simulink model "Thirtybussys1"  (R2021a)
settings: Solver=VariableStepAuto  StartTime=0.0  StopTime=4.0  RelTol=1e-3
libraries: spsFourierLib x60, spsThreePhaseSeriesRLCBranchLib x41, spsThreePhaseVIMeasurementLib x30, spsThreePhaseSeriesRLCLoadLib x21, spsThreePhaseSourceLib x6, spsThreePhaseTransformerTwoWindingsLib x6, spsThreePhaseFaultLib x2, spspowerguiLib x1
(part 1 of 2)
settings Model: Creator=sariy sh  LastModifiedBy=Maruf
settings SolverCC: AlgebraicLoopSolver=TrustRegion
settings DataIOCC: ReturnWorkspaceOutputs=off
settings DebuggingCC: SFMachineParentedDataDiag=warning  ArithmeticOperatorsInVariantConditions=warning
settings SFSimCC: SimUseLocalCustomCode=off  CustomCodeUndefinedFunction=UseInterfaceOnly
settings RTWCC: RTWUseLocalCustomCode=off
settings CodeAppCC: StateflowObjectComments=on
settings SimscapeCC: SimscapeNormalizeSystem=off

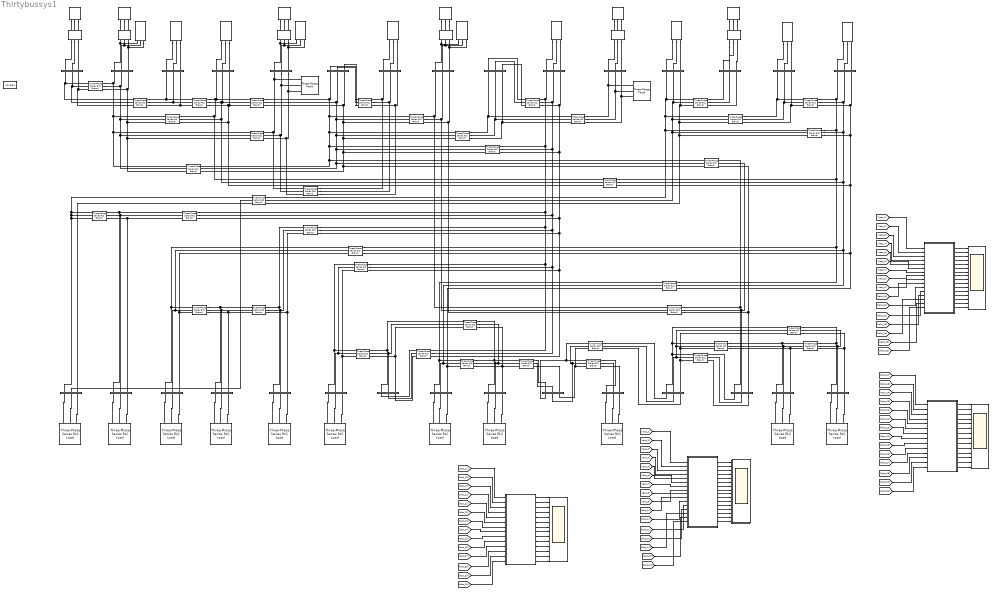
== system Thirtybussys1 ==
  3-Phase Fault : spsThreePhaseFaultLib/Three-Phase Fault  InitialStates=0  FaultA=on  FaultB=on  FaultC=on  GroundFault=on  SwitchTimes=[2.1 3.1]  External=off  SwitchStatus=NaN  FaultResistance=0.01  GroundResistance=0.001  SnubberResistance=1e6  SnubberCapacitance=inf  Measurements=Fault currents
  3-Phase Fault1 : spsThreePhaseFaultLib/Three-Phase Fault  InitialStates=0  FaultA=on  FaultB=on  FaultC=on  GroundFault=on  SwitchTimes=[2.1 3.1]  External=off  SwitchStatus=NaN  FaultResistance=0.01  GroundResistance=0.001  SnubberResistance=1e6  SnubberCapacitance=inf  Measurements=Fault currents
  Bus 1 : spsThreePhaseVIMeasurementLib/Three-Phase V-I Measurement  VoltageMeasurement=phase-to-ground  SetLabelV=on  LabelV=Vabc_1  Vpu=on  VpuLL=off  CurrentMeasurement=yes  SetLabelI=on  LabelI=Iabc_1  Ipu=on  Pbase=100e6  Vbase=500e3  OutputType=Complex  PhasorSimulation=off  PSBequivalent=0
  Bus 10 : spsThreePhaseVIMeasurementLib/Three-Phase V-I Measurement  VoltageMeasurement=phase-to-ground  SetLabelV=on  LabelV=Vabc_10  Vpu=on  VpuLL=off  CurrentMeasurement=yes  SetLabelI=on  LabelI=Iabc_10  Ipu=on  Pbase=100e6  Vbase=500e3  OutputType=Complex  PhasorSimulation=off  PSBequivalent=0
  Bus 11 : spsThreePhaseVIMeasurementLib/Three-Phase V-I Measurement  VoltageMeasurement=phase-to-ground  SetLabelV=on  LabelV=Vabc_11  Vpu=on  VpuLL=off  CurrentMeasurement=yes  SetLabelI=on  LabelI=Iabc_11  Ipu=on  Pbase=100e6  Vbase=500e3  OutputType=Complex  PhasorSimulation=off  PSBequivalent=0
  Bus 12 : spsThreePhaseVIMeasurementLib/Three-Phase V-I Measurement  VoltageMeasurement=phase-to-ground  SetLabelV=on  LabelV=Vabc_12  Vpu=on  VpuLL=off  CurrentMeasurement=yes  SetLabelI=on  LabelI=Iabc_12  Ipu=on  Pbase=100e6  Vbase=500e3  OutputType=Complex  PhasorSimulation=off  PSBequivalent=0
  Bus 13 : spsThreePhaseVIMeasurementLib/Three-Phase V-I Measurement  VoltageMeasurement=phase-to-ground  SetLabelV=on  LabelV=Vabc_13  Vpu=on  VpuLL=off  CurrentMeasurement=yes  SetLabelI=on  LabelI=Iabc_13  Ipu=on  Pbase=100e6  Vbase=500e3  OutputType=Complex  PhasorSimulation=off  PSBequivalent=0
  Bus 14 : spsThreePhaseVIMeasurementLib/Three-Phase V-I Measurement  VoltageMeasurement=phase-to-ground  SetLabelV=on  LabelV=Vabc_14  Vpu=on  VpuLL=off  CurrentMeasurement=yes  SetLabelI=on  LabelI=Iabc_14  Ipu=on  Pbase=100e6  Vbase=500e3  OutputType=Complex  PhasorSimulation=off  PSBequivalent=0
  Bus 15 : spsThreePhaseVIMeasurementLib/Three-Phase V-I Measurement  VoltageMeasurement=phase-to-ground  SetLabelV=on  LabelV=Vabc_15  Vpu=on  VpuLL=off  CurrentMeasurement=yes  SetLabelI=on  LabelI=Iabc_15  Ipu=on  Pbase=100e6  Vbase=500e3  OutputType=Complex  PhasorSimulation=off  PSBequivalent=0
  Bus 16 : spsThreePhaseVIMeasurementLib/Three-Phase V-I Measurement  VoltageMeasurement=phase-to-ground  SetLabelV=on  LabelV=Vabc_16  Vpu=on  VpuLL=off  CurrentMeasurement=yes  SetLabelI=on  LabelI=Iabc_16  Ipu=on  Pbase=100e6  Vbase=500e3  OutputType=Complex  PhasorSimulation=off  PSBequivalent=0
  Bus 17 : spsThreePhaseVIMeasurementLib/Three-Phase V-I Measurement  VoltageMeasurement=phase-to-ground  SetLabelV=on  LabelV=Vabc_17  Vpu=on  VpuLL=off  CurrentMeasurement=yes  SetLabelI=on  LabelI=Iabc_17  Ipu=on  Pbase=100e6  Vbase=500e3  OutputType=Complex  PhasorSimulation=off  PSBequivalent=0
  Bus 18 : spsThreePhaseVIMeasurementLib/Three-Phase V-I Measurement  VoltageMeasurement=phase-to-ground  SetLabelV=on  LabelV=Vabc_18  Vpu=on  VpuLL=off  CurrentMeasurement=yes  SetLabelI=on  LabelI=Iabc_18  Ipu=on  Pbase=100e6  Vbase=500e3  OutputType=Complex  PhasorSimulation=off  PSBequivalent=0
  Bus 19 : spsThreePhaseVIMeasurementLib/Three-Phase V-I Measurement  VoltageMeasurement=phase-to-ground  SetLabelV=on  LabelV=Vabc_19  Vpu=on  VpuLL=off  CurrentMeasurement=yes  SetLabelI=on  LabelI=Iabc_19  Ipu=on  Pbase=100e6  Vbase=500e3  OutputType=Complex  PhasorSimulation=off  PSBequivalent=0
  Bus 2 : spsThreePhaseVIMeasurementLib/Three-Phase V-I Measurement  VoltageMeasurement=phase-to-ground  SetLabelV=on  LabelV=Vabc_2  Vpu=on  VpuLL=off  CurrentMeasurement=yes  SetLabelI=on  LabelI=Iabc_2  Ipu=on  Pbase=100e6  Vbase=500e3  OutputType=Complex  PhasorSimulation=off  PSBequivalent=0
  Bus 20 : spsThreePhaseVIMeasurementLib/Three-Phase V-I Measurement  VoltageMeasurement=phase-to-ground  SetLabelV=on  LabelV=Vabc_20  Vpu=on  VpuLL=off  CurrentMeasurement=yes  SetLabelI=on  LabelI=Iabc_20  Ipu=on  Pbase=100e6  Vbase=500e3  OutputType=Complex  PhasorSimulation=off  PSBequivalent=0
  Bus 21 : spsThreePhaseVIMeasurementLib/Three-Phase V-I Measurement  VoltageMeasurement=phase-to-ground  SetLabelV=on  LabelV=Vabc_21  Vpu=on  VpuLL=off  CurrentMeasurement=yes  SetLabelI=on  LabelI=Iabc_21  Ipu=on  Pbase=100e6  Vbase=500e3  OutputType=Complex  PhasorSimulation=off  PSBequivalent=0
  Bus 22 : spsThreePhaseVIMeasurementLib/Three-Phase V-I Measurement  VoltageMeasurement=phase-to-ground  SetLabelV=on  LabelV=Vabc_22  Vpu=on  VpuLL=off  CurrentMeasurement=yes  SetLabelI=on  LabelI=Iabc_22  Ipu=on  Pbase=100e6  Vbase=500e3  OutputType=Complex  PhasorSimulation=off  PSBequivalent=0
  Bus 23 : spsThreePhaseVIMeasurementLib/Three-Phase V-I Measurement  VoltageMeasurement=phase-to-ground  SetLabelV=on  LabelV=Vabc_23  Vpu=on  VpuLL=off  CurrentMeasurement=yes  SetLabelI=on  LabelI=Iabc_23  Ipu=on  Pbase=100e6  Vbase=500e3  OutputType=Complex  PhasorSimulation=off  PSBequivalent=0
  Bus 24 : spsThreePhaseVIMeasurementLib/Three-Phase V-I Measurement  VoltageMeasurement=phase-to-ground  SetLabelV=on  LabelV=Vabc_24  Vpu=on  VpuLL=off  CurrentMeasurement=yes  SetLabelI=on  LabelI=Iabc_24  Ipu=on  Pbase=100e6  Vbase=500e3  OutputType=Complex  PhasorSimulation=off  PSBequivalent=0
  Bus 25 : spsThreePhaseVIMeasurementLib/Three-Phase V-I Measurement  VoltageMeasurement=phase-to-ground  SetLabelV=on  LabelV=Vabc_25  Vpu=on  VpuLL=off  CurrentMeasurement=yes  SetLabelI=on  LabelI=Iabc_25  Ipu=on  Pbase=100e6  Vbase=500e3  OutputType=Complex  PhasorSimulation=off  PSBequivalent=0
  Bus 26 : spsThreePhaseVIMeasurementLib/Three-Phase V-I Measurement  VoltageMeasurement=phase-to-ground  SetLabelV=on  LabelV=Vabc_26  Vpu=on  VpuLL=off  CurrentMeasurement=yes  SetLabelI=on  LabelI=Iabc_26  Ipu=on  Pbase=100e6  Vbase=500e3  OutputType=Complex  PhasorSimulation=off  PSBequivalent=0
  Bus 27 : spsThreePhaseVIMeasurementLib/Three-Phase V-I Measurement  VoltageMeasurement=phase-to-ground  SetLabelV=on  LabelV=Vabc_27  Vpu=on  VpuLL=off  CurrentMeasurement=yes  SetLabelI=on  LabelI=Iabc_27  Ipu=on  Pbase=100e6  Vbase=500e3  OutputType=Complex  PhasorSimulation=off  PSBequivalent=0
  Bus 28 : spsThreePhaseVIMeasurementLib/Three-Phase V-I Measurement  VoltageMeasurement=phase-to-ground  SetLabelV=on  LabelV=Vabc_28  Vpu=on  VpuLL=off  CurrentMeasurement=yes  SetLabelI=on  LabelI=Iabc_28  Ipu=on  Pbase=100e6  Vbase=500e3  OutputType=Complex  PhasorSimulation=off  PSBequivalent=0
  Bus 29 : spsThreePhaseVIMeasurementLib/Three-Phase V-I Measurement  VoltageMeasurement=phase-to-ground  SetLabelV=on  LabelV=Vabc_29  Vpu=on  VpuLL=off  CurrentMeasurement=yes  SetLabelI=on  LabelI=Iabc_29  Ipu=on  Pbase=100e6  Vbase=500e3  OutputType=Complex  PhasorSimulation=off  PSBequivalent=0
  Bus 3 : spsThreePhaseVIMeasurementLib/Three-Phase V-I Measurement  VoltageMeasurement=phase-to-ground  SetLabelV=on  LabelV=Vabc_3  Vpu=on  VpuLL=off  CurrentMeasurement=yes  SetLabelI=on  LabelI=Iabc_3  Ipu=on  Pbase=100e6  Vbase=500e3  OutputType=Complex  PhasorSimulation=off  PSBequivalent=0
  Bus 30 : spsThreePhaseVIMeasurementLib/Three-Phase V-I Measurement  VoltageMeasurement=phase-to-ground  SetLabelV=on  LabelV=Vabc_30  Vpu=on  VpuLL=off  CurrentMeasurement=yes  SetLabelI=on  LabelI=Iabc_30  Ipu=on  Pbase=100e6  Vbase=500e3  OutputType=Complex  PhasorSimulation=off  PSBequivalent=0
  Bus 4 : spsThreePhaseVIMeasurementLib/Three-Phase V-I Measurement  VoltageMeasurement=phase-to-ground  SetLabelV=on  LabelV=Vabc_4  Vpu=on  VpuLL=off  CurrentMeasurement=yes  SetLabelI=on  LabelI=Iabc_4  Ipu=on  Pbase=100e6  Vbase=500e3  OutputType=Complex  PhasorSimulation=off  PSBequivalent=0
  Bus 5 : spsThreePhaseVIMeasurementLib/Three-Phase V-I Measurement  VoltageMeasurement=phase-to-ground  SetLabelV=on  LabelV=Vabc_5  Vpu=on  VpuLL=off  CurrentMeasurement=yes  SetLabelI=on  LabelI=Iabc_5  Ipu=on  Pbase=100e6  Vbase=500e3  OutputType=Complex  PhasorSimulation=off  PSBequivalent=0
  Bus 6 : spsThreePhaseVIMeasurementLib/Three-Phase V-I Measurement  VoltageMeasurement=phase-to-ground  SetLabelV=on  LabelV=Vabc_6  Vpu=on  VpuLL=off  CurrentMeasurement=yes  SetLabelI=on  LabelI=Iabc_6  Ipu=on  Pbase=100e6  Vbase=500e3  OutputType=Complex  PhasorSimulation=off  PSBequivalent=0
  Bus 7 : spsThreePhaseVIMeasurementLib/Three-Phase V-I Measurement  VoltageMeasurement=phase-to-ground  SetLabelV=on  LabelV=Vabc_7  Vpu=on  VpuLL=off  CurrentMeasurement=yes  SetLabelI=on  LabelI=Iabc_7  Ipu=on  Pbase=100e6  Vbase=500e3  OutputType=Complex  PhasorSimulation=off  PSBequivalent=0
  Bus 8 : spsThreePhaseVIMeasurementLib/Three-Phase V-I Measurement  VoltageMeasurement=phase-to-ground  SetLabelV=on  LabelV=Vabc_8  Vpu=on  VpuLL=off  CurrentMeasurement=yes  SetLabelI=on  LabelI=Iabc_8  Ipu=on  Pbase=100e6  Vbase=500e3  OutputType=Complex  PhasorSimulation=off  PSBequivalent=0
  Bus 9 : spsThreePhaseVIMeasurementLib/Three-Phase V-I Measurement  VoltageMeasurement=phase-to-ground  SetLabelV=on  LabelV=Vabc_9  Vpu=on  VpuLL=off  CurrentMeasurement=yes  SetLabelI=on  LabelI=Iabc_9  Ipu=on  Pbase=100e6  Vbase=500e3  OutputType=Complex  PhasorSimulation=off  PSBequivalent=0
  Gen1 : spsThreePhaseSourceLib/Three-Phase Source  InternalConnection=Yg  VoltagePhases=off  Voltage=1.06  PhaseAngle=0  Voltage_phases=[25e3 25e3 25e3]/sqrt(3)  PhaseAngles_phases=[0 -120 +120]  Frequency=50  NonIdealSource=on  SpecifyImpedance=on  Resistance=0.8929  Inductance=16.58e-3  ShortCircuitLevel=100e6  BaseVoltage=1  XRratio=1  BusType=swing  Pref=10e3  Qref=0  Prefabc=[10e3, 10e3, 10e3]  Qrefabc=[0, 0, 0]  Qmin=-inf  Qmax=inf
  Gen2 : spsThreePhaseSourceLib/Three-Phase Source  InternalConnection=Yg  VoltagePhases=off  Voltage=1.045  PhaseAngle=0  Voltage_phases=[25e3 25e3 25e3]/sqrt(3)  PhaseAngles_phases=[0 -120 +120]  Frequency=50  NonIdealSource=on  SpecifyImpedance=on  Resistance=0.8929  Inductance=16.58e-3  ShortCircuitLevel=100e6  BaseVoltage=1  XRratio=1  BusType=PQ  Pref=0.4  Qref=0.5  Prefabc=[10e3, 10e3, 10e3]  Qrefabc=[0, 0, 0]  Qmin=-inf  Qmax=inf
  Gen3 : spsThreePhaseSourceLib/Three-Phase Source  InternalConnection=Yg  VoltagePhases=off  Voltage=1.010  PhaseAngle=0  Voltage_phases=[25e3 25e3 25e3]/sqrt(3)  PhaseAngles_phases=[0 -120 +120]  Frequency=50  NonIdealSource=on  SpecifyImpedance=on  Resistance=0.8929  Inductance=16.58e-3  ShortCircuitLevel=100e6  BaseVoltage=1  XRratio=1  BusType=PV  Pref=0.37  Qref=0  Prefabc=[10e3, 10e3, 10e3]  Qrefabc=[0, 0, 0]  Qmin=-0.15  Qmax=0.625
  Gen4 : spsThreePhaseSourceLib/Three-Phase Source  InternalConnection=Yg  VoltagePhases=off  Voltage=1.010  PhaseAngle=0  Voltage_phases=[25e3 25e3 25e3]/sqrt(3)  PhaseAngles_phases=[0 -120 +120]  Frequency=50  NonIdealSource=on  SpecifyImpedance=on  Resistance=0.8929  Inductance=16.58e-3  ShortCircuitLevel=100e6  BaseVoltage=1  XRratio=1  BusType=PV  Pref=0.373  Qref=0  Prefabc=[10e3, 10e3, 10e3]  Qrefabc=[0, 0, 0]  Qmin=-0.15  Qmax=0.50
  Gen5 : spsThreePhaseSourceLib/Three-Phase Source  InternalConnection=Yg  VoltagePhases=off  Voltage=1.082  PhaseAngle=0  Voltage_phases=[25e3 25e3 25e3]/sqrt(3)  PhaseAngles_phases=[0 -120 +120]  Frequency=50  NonIdealSource=on  SpecifyImpedance=on  Resistance=0.8929  Inductance=16.58e-3  ShortCircuitLevel=100e6  BaseVoltage=1  XRratio=1  BusType=PV  Pref=0.162  Qref=0  Prefabc=[10e3, 10e3, 10e3]  Qrefabc=[0, 0, 0]  Qmin=-0.10  Qmax=0.40
  Gen6 : spsThreePhaseSourceLib/Three-Phase Source  InternalConnection=Yg  VoltagePhases=off  Voltage=1.071  PhaseAngle=0  Voltage_phases=[25e3 25e3 25e3]/sqrt(3)  PhaseAngles_phases=[0 -120 +120]  Frequency=50  NonIdealSource=on  SpecifyImpedance=on  Resistance=0.8929  Inductance=16.58e-3  ShortCircuitLevel=100e6  BaseVoltage=1  XRratio=1  BusType=PV  Pref=0.106  Qref=0  Prefabc=[10e3, 10e3, 10e3]  Qrefabc=[0, 0, 0]  Qmin=-0.15  Qmax=0.45
  Scope1 : Scope  NumInputPorts=14
  Scope2 : Scope  NumInputPorts=16
  Scope3 : Scope  NumInputPorts=16
  Scope4 : Scope  NumInputPorts=14
  Scope5 : Scope  NumInputPorts=16
  Subsystem : Subsystem
  Subsystem1 : Subsystem
  Subsystem2 : Subsystem
  Subsystem3 : Subsystem
  Three-Phase Series RLC Branch : spsThreePhaseSeriesRLCBranchLib/Three-Phase Series RLC Branch  LConnTagsString=A|B|C  RConnTagsString=A|B|C  BranchType=RLC  Resistance=0.0192  Inductance=0.0575/(2*pi*50)  Capacitance=1/0.0264/(2*pi*50)  Measurements=None
  Three-Phase Series RLC Branch1 : spsThreePhaseSeriesRLCBranchLib/Three-Phase Series RLC Branch  LConnTagsString=A|B|C  RConnTagsString=A|B|C  BranchType=RLC  Resistance=0.0452  Inductance=0.1652/(2*pi*50)  Capacitance=1/0.0204/(2*pi*50)  Measurements=None
  Three-Phase Series RLC Branch10 : spsThreePhaseSeriesRLCBranchLib/Three-Phase Series RLC Branch  LConnTagsString=A|B|C  RConnTagsString=A|B|C  BranchType=L  Resistance=0  Inductance=0.2080/(2*pi*50)  Capacitance=0  Measurements=None
  Three-Phase Series RLC Branch11 : spsThreePhaseSeriesRLCBranchLib/Three-Phase Series RLC Branch  LConnTagsString=A|B|C  RConnTagsString=A|B|C  BranchType=L  Resistance=1  Inductance=0.1100/(2*pi*50)  Capacitance=1e-6  Measurements=None
  Three-Phase Series RLC Branch12 : spsThreePhaseSeriesRLCBranchLib/Three-Phase Series RLC Branch  LConnTagsString=A|B|C  RConnTagsString=A|B|C  BranchType=L  Resistance=1  Inductance=0.5560/(2*pi*50)  Capacitance=1e-6  Measurements=None
  Three-Phase Series RLC Branch13 : spsThreePhaseSeriesRLCBranchLib/Three-Phase Series RLC Branch  LConnTagsString=A|B|C  RConnTagsString=A|B|C  BranchType=L  Resistance=1  Inductance=0.2080/(2*pi*50)  Capacitance=1e-6  Measurements=None
  Three-Phase Series RLC Branch14 : spsThreePhaseSeriesRLCBranchLib/Three-Phase Series RLC Branch  LConnTagsString=A|B|C  RConnTagsString=A|B|C  BranchType=L  Resistance=1  Inductance=0.1400/(2*pi*50)  Capacitance=1e-6  Measurements=None
  Three-Phase Series RLC Branch15 : spsThreePhaseSeriesRLCBranchLib/Three-Phase Series RLC Branch  LConnTagsString=A|B|C  RConnTagsString=A|B|C  BranchType=RL  Resistance=0.1231  Inductance=0.2559/(2*pi*50)  Capacitance=1e-6  Measurements=None
  Three-Phase Series RLC Branch16 : spsThreePhaseSeriesRLCBranchLib/Three-Phase Series RLC Branch  LConnTagsString=A|B|C  RConnTagsString=A|B|C  BranchType=RL  Resistance=0.2210  Inductance=0.1997/(2*pi*50)  Capacitance=1e-6  Measurements=None
  Three-Phase Series RLC Branch17 : spsThreePhaseSeriesRLCBranchLib/Three-Phase Series RLC Branch  LConnTagsString=A|B|C  RConnTagsString=A|B|C  BranchType=L  Resistance=1  Inductance=0.2560/(2*pi*50)  Capacitance=1e-6  Measurements=None
  Three-Phase Series RLC Branch18 : spsThreePhaseSeriesRLCBranchLib/Three-Phase Series RLC Branch  LConnTagsString=A|B|C  RConnTagsString=A|B|C  BranchType=RL  Resistance=0.0945  Inductance=0.1987/(2*pi*50)  Capacitance=1e-6  Measurements=None
  Three-Phase Series RLC Branch19 : spsThreePhaseSeriesRLCBranchLib/Three-Phase Series RLC Branch  LConnTagsString=A|B|C  RConnTagsString=A|B|C  BranchType=RLC  Resistance=0.0524  Inductance=0.1923/(2*pi*50)  Capacitance=1e-6  Measurements=None
  Three-Phase Series RLC Branch2 : spsThreePhaseSeriesRLCBranchLib/Three-Phase Series RLC Branch  LConnTagsString=A|B|C  RConnTagsString=A|B|C  BranchType=RLC  Resistance=0.0132  Inductance=0.0379/(2*pi*50)  Capacitance=1/0.0042/(2*pi*50)  Measurements=None
  Three-Phase Series RLC Branch20 : spsThreePhaseSeriesRLCBranchLib/Three-Phase Series RLC Branch  LConnTagsString=A|B|C  RConnTagsString=A|B|C  BranchType=RL  Resistance=0.0324  Inductance=0.0845/(2*pi*50)  Capacitance=1e-6  Measurements=None
  Three-Phase Series RLC Branch21 : spsThreePhaseSeriesRLCBranchLib/Three-Phase Series RLC Branch  LConnTagsString=A|B|C  RConnTagsString=A|B|C  BranchType=RL  Resistance=0.1063  Inductance=0.2185/(2*pi*50)  Capacitance=1e-6  Measurements=None
  Three-Phase Series RLC Branch22 : spsThreePhaseSeriesRLCBranchLib/Three-Phase Series RLC Branch  LConnTagsString=A|B|C  RConnTagsString=A|B|C  BranchType=RL  Resistance=0.0639  Inductance=0.1292/(2*pi*50)  Capacitance=1e-6  Measurements=None
  Three-Phase Series RLC Branch23 : spsThreePhaseSeriesRLCBranchLib/Three-Phase Series RLC Branch  LConnTagsString=A|B|C  RConnTagsString=A|B|C  BranchType=RL  Resistance=0.0340  Inductance=0.0680/(2*pi*50)  Capacitance=1e-6  Measurements=None
  Three-Phase Series RLC Branch24 : spsThreePhaseSeriesRLCBranchLib/Three-Phase Series RLC Branch  LConnTagsString=A|B|C  RConnTagsString=A|B|C  BranchType=RL  Resistance=0.0936  Inductance=0.2090/(2*pi*50)  Capacitance=1e-6  Measurements=None
  Three-Phase Series RLC Branch25 : spsThreePhaseSeriesRLCBranchLib/Three-Phase Series RLC Branch  LConnTagsString=A|B|C  RConnTagsString=A|B|C  BranchType=RL  Resistance=0.0348  Inductance=0.0749/(2*pi*50)  Capacitance=1e-6  Measurements=None
  Three-Phase Series RLC Branch26 : spsThreePhaseSeriesRLCBranchLib/Three-Phase Series RLC Branch  LConnTagsString=A|B|C  RConnTagsString=A|B|C  BranchType=RL  Resistance=0.0116  Inductance=0.0236/(2*pi*50)  Capacitance=1e-6  Measurements=None
  Three-Phase Series RLC Branch27 : spsThreePhaseSeriesRLCBranchLib/Three-Phase Series RLC Branch  LConnTagsString=A|B|C  RConnTagsString=A|B|C  BranchType=RL  Resistance=0.0727  Inductance=0.1499/(2*pi*50)  Capacitance=1e-6  Measurements=None
  Three-Phase Series RLC Branch28 : spsThreePhaseSeriesRLCBranchLib/Three-Phase Series RLC Branch  LConnTagsString=A|B|C  RConnTagsString=A|B|C  BranchType=RL  Resistance=0.1000  Inductance=0.2020/(2*pi*50)  Capacitance=1e-6  Measurements=None
  Three-Phase Series RLC Branch29 : spsThreePhaseSeriesRLCBranchLib/Three-Phase Series RLC Branch  LConnTagsString=A|B|C  RConnTagsString=A|B|C  BranchType=RL  Resistance=0.1150  Inductance=0.1790/(2*pi*50)  Capacitance=1e-6  Measurements=None
  Three-Phase Series RLC Branch3 : spsThreePhaseSeriesRLCBranchLib/Three-Phase Series RLC Branch  LConnTagsString=A|B|C  RConnTagsString=A|B|C  BranchType=RLC  Resistance=0.0570  Inductance=0.1737/(2*pi*50)  Capacitance=1/0.0184/(2*pi*50)  Measurements=None
  Three-Phase Series RLC Branch30 : spsThreePhaseSeriesRLCBranchLib/Three-Phase Series RLC Branch  LConnTagsString=A|B|C  RConnTagsString=A|B|C  BranchType=RL  Resistance=0.1320  Inductance=0.2700/(2*pi*50)  Capacitance=1e-6  Measurements=None
  Three-Phase Series RLC Branch31 : spsThreePhaseSeriesRLCBranchLib/Three-Phase Series RLC Branch  LConnTagsString=A|B|C  RConnTagsString=A|B|C  BranchType=RL  Resistance=0.1885  Inductance=0.3292/(2*pi*50)  Capacitance=1e-6  Measurements=None
  Three-Phase Series RLC Branch32 : spsThreePhaseSeriesRLCBranchLib/Three-Phase Series RLC Branch  LConnTagsString=A|B|C  RConnTagsString=A|B|C  BranchType=RL  Resistance=0.2544  Inductance=0.3800/(2*pi*50)  Capacitance=1e-6  Measurements=None
  Three-Phase Series RLC Branch33 : spsThreePhaseSeriesRLCBranchLib/Three-Phase Series RLC Branch  LConnTagsString=A|B|C  RConnTagsString=A|B|C  BranchType=RL  Resistance=0.1093  Inductance=0.2087/(2*pi*50)  Capacitance=1e-6  Measurements=None
  Three-Phase Series RLC Branch34 : spsThreePhaseSeriesRLCBranchLib/Three-Phase Series RLC Branch  LConnTagsString=A|B|C  RConnTagsString=A|B|C  BranchType=RL  Resistance=0.2198  Inductance=0.4153/(2*pi*50)  Capacitance=1e-6  Measurements=None
  Three-Phase Series RLC Branch35 : spsThreePhaseSeriesRLCBranchLib/Three-Phase Series RLC Branch  LConnTagsString=A|B|C  RConnTagsString=A|B|C  BranchType=RL  Resistance=0.3202  Inductance=0.6027/(2*pi*50)  Capacitance=1e-6  Measurements=None
  Three-Phase Series RLC Branch36 : spsThreePhaseSeriesRLCBranchLib/Three-Phase Series RLC Branch  LConnTagsString=A|B|C  RConnTagsString=A|B|C  BranchType=L  Resistance=1  Inductance=0.3960/(2*pi*50)  Capacitance=1e-6  Measurements=None
  Three-Phase Series RLC Branch37 : spsThreePhaseSeriesRLCBranchLib/Three-Phase Series RLC Branch  LConnTagsString=A|B|C  RConnTagsString=A|B|C  BranchType=RLC  Resistance=0.0169  Inductance=0.0599/(2*pi*50)  Capacitance=1/0.0065/(2*pi*50)  Measurements=None
  Three-Phase Series RLC Branch38 : spsThreePhaseSeriesRLCBranchLib/Three-Phase Series RLC Branch  LConnTagsString=A|B|C  RConnTagsString=A|B|C  BranchType=RLC  Resistance=0.0636  Inductance=0.2000/(2*pi*50)  Capacitance=1/0.0214/(2*pi*50)  Measurements=None
  Three-Phase Series RLC Branch39 : spsThreePhaseSeriesRLCBranchLib/Three-Phase Series RLC Branch  LConnTagsString=A|B|C  RConnTagsString=A|B|C  BranchType=RL  Resistance=0.0662  Inductance=0.1304/(2*pi*50)  Capacitance=1e-6  Measurements=None
  Three-Phase Series RLC Branch4 : spsThreePhaseSeriesRLCBranchLib/Three-Phase Series RLC Branch  LConnTagsString=A|B|C  RConnTagsString=A|B|C  BranchType=RLC  Resistance=0.0472  Inductance=0.1983/(2*pi*50)  Capacitance=1/0.0209/(2*pi*50)  Measurements=None
  Three-Phase Series RLC Branch40 : spsThreePhaseSeriesRLCBranchLib/Three-Phase Series RLC Branch  LConnTagsString=A|B|C  RConnTagsString=A|B|C  BranchType=RL  Resistance=0.2399  Inductance=0.4533/(2*pi*50)  Capacitance=1e-6  Measurements=None
  Three-Phase Series RLC Branch5 : spsThreePhaseSeriesRLCBranchLib/Three-Phase Series RLC Branch  LConnTagsString=A|B|C  RConnTagsString=A|B|C  BranchType=RLC  Resistance=0.0581  Inductance=0.1763/(2*pi*50)  Capacitance=1/0.0187/(2*pi*50)  Measurements=None
  Three-Phase Series RLC Branch6 : spsThreePhaseSeriesRLCBranchLib/Three-Phase Series RLC Branch  LConnTagsString=A|B|C  RConnTagsString=A|B|C  BranchType=RLC  Resistance=0.0119  Inductance=0.0414/(2*pi*50)  Capacitance=1/0.0045/(2*pi*50)  Measurements=None
  Three-Phase Series RLC Branch7 : spsThreePhaseSeriesRLCBranchLib/Three-Phase Series RLC Branch  LConnTagsString=A|B|C  RConnTagsString=A|B|C  BranchType=RLC  Resistance=0.0267  Inductance=0.0820/(2*pi*50)  Capacitance=1/0.0085/(2*pi*50)  Measurements=None
  Three-Phase Series RLC Branch8 : spsThreePhaseSeriesRLCBranchLib/Three-Phase Series RLC Branch  LConnTagsString=A|B|C  RConnTagsString=A|B|C  BranchType=RLC  Resistance=0.0460  Inductance=0.1160/(2*pi*50)  Capacitance=1/0.0102/(2*pi*50)  Measurements=None
  Three-Phase Series RLC Branch9 : spsThreePhaseSeriesRLCBranchLib/Three-Phase Series RLC Branch  LConnTagsString=A|B|C  RConnTagsString=A|B|C  BranchType=RLC  Resistance=0.0120  Inductance=0.0420/(2*pi*50)  Capacitance=1/0.0045/(2*pi*50)  Measurements=None
  Three-Phase Series RLC Load : spsThreePhaseSeriesRLCLoadLib/Three-Phase Series RLC Load  LConnTagsString=A|B|C  Configuration=Y (grounded)  NominalVoltage=1  Vabc=[1e3 1e3 1e3]  Vabcp=[1e3 1e3 1e3]  NominalFrequency=50  UnbalancedPower=off  ActivePower=0.217  InductivePower=0.127  CapacitivePower=0  Pabc=[10e3 9e3 11e3]  QLabc=[100 90 110]  QCabc=[100 90 110]  Pabcp=[10e3 9e3 11e3]  QLabcp=[100 90 110]  QCabcp=[100 90 110]  Measurements=None  LoadType=constant Z
  Three-Phase Series RLC Load1 : spsThreePhaseSeriesRLCLoadLib/Three-Phase Series RLC Load  LConnTagsString=A|B|C  Configuration=Y (grounded)  NominalVoltage=1  Vabc=[1e3 1e3 1e3]  Vabcp=[1e3 1e3 1e3]  NominalFrequency=50  UnbalancedPower=off  ActivePower=0.024  InductivePower=0.012  CapacitivePower=0  Pabc=[10e3 9e3 11e3]  QLabc=[100 90 110]  QCabc=[100 90 110]  Pabcp=[10e3 9e3 11e3]  QLabcp=[100 90 110]  QCabcp=[100 90 110]  Measurements=None  LoadType=constant Z
  Three-Phase Series RLC Load10 : spsThreePhaseSeriesRLCLoadLib/Three-Phase Series RLC Load  LConnTagsString=A|B|C  Configuration=Y (grounded)  NominalVoltage=1  Vabc=[1e3 1e3 1e3]  Vabcp=[1e3 1e3 1e3]  NominalFrequency=50  UnbalancedPower=off  ActivePower=0.062  InductivePower=0.016  CapacitivePower=0  Pabc=[10e3 9e3 11e3]  QLabc=[100 90 110]  QCabc=[100 90 110]  Pabcp=[10e3 9e3 11e3]  QLabcp=[100 90 110]  QCabcp=[100 90 110]  Measurements=None  LoadType=constant Z
  Three-Phase Series RLC Load11 : spsThreePhaseSeriesRLCLoadLib/Three-Phase Series RLC Load  LConnTagsString=A|B|C  Configuration=Y (grounded)  NominalVoltage=1  Vabc=[1e3 1e3 1e3]  Vabcp=[1e3 1e3 1e3]  NominalFrequency=50  UnbalancedPower=off  ActivePower=0.082  InductivePower=0.025  CapacitivePower=0  Pabc=[10e3 9e3 11e3]  QLabc=[100 90 110]  QCabc=[100 90 110]  Pabcp=[10e3 9e3 11e3]  QLabcp=[100 90 110]  QCabcp=[100 90 110]  Measurements=None  LoadType=constant Z
  Three-Phase Series RLC Load12 : spsThreePhaseSeriesRLCLoadLib/Three-Phase Series RLC Load  LConnTagsString=A|B|C  Configuration=Y (grounded)  NominalVoltage=1  Vabc=[1e3 1e3 1e3]  Vabcp=[1e3 1e3 1e3]  NominalFrequency=50  UnbalancedPower=off  ActivePower=0.3  InductivePower=0.3  CapacitivePower=0  Pabc=[10e3 9e3 11e3]  QLabc=[100 90 110]  QCabc=[100 90 110]  Pabcp=[10e3 9e3 11e3]  QLabcp=[100 90 110]  QCabcp=[100 90 110]  Measurements=None  LoadType=constant Z
  Three-Phase Series RLC Load13 : spsThreePhaseSeriesRLCLoadLib/Three-Phase Series RLC Load  LConnTagsString=A|B|C  Configuration=Y (grounded)  NominalVoltage=1  Vabc=[1e3 1e3 1e3]  Vabcp=[1e3 1e3 1e3]  NominalFrequency=50  UnbalancedPower=off  ActivePower=0.032  InductivePower=0.009  CapacitivePower=0  Pabc=[10e3 9e3 11e3]  QLabc=[100 90 110]  QCabc=[100 90 110]  Pabcp=[10e3 9e3 11e3]  QLabcp=[100 90 110]  QCabcp=[100 90 110]  Measurements=None  LoadType=constant Z
  Three-Phase Series RLC Load14 : spsThreePhaseSeriesRLCLoadLib/Three-Phase Series RLC Load  LConnTagsString=A|B|C  Configuration=Y (grounded)  NominalVoltage=1  Vabc=[1e3 1e3 1e3]  Vabcp=[1e3 1e3 1e3]  NominalFrequency=50  UnbalancedPower=off  ActivePower=0.095  InductivePower=0.034  CapacitivePower=0  Pabc=[10e3 9e3 11e3]  QLabc=[100 90 110]  QCabc=[100 90 110]  Pabcp=[10e3 9e3 11e3]  QLabcp=[100 90 110]  QCabcp=[100 90 110]  Measurements=None  LoadType=constant Z
  Three-Phase Series RLC Load15 : spsThreePhaseSeriesRLCLoadLib/Three-Phase Series RLC Load  LConnTagsString=A|B|C  Configuration=Y (grounded)  NominalVoltage=1  Vabc=[1e3 1e3 1e3]  Vabcp=[1e3 1e3 1e3]  NominalFrequency=50  UnbalancedPower=off  ActivePower=0.022  InductivePower=0.007  CapacitivePower=0  Pabc=[10e3 9e3 11e3]  QLabc=[100 90 110]  QCabc=[100 90 110]  Pabcp=[10e3 9e3 11e3]  QLabcp=[100 90 110]  QCabcp=[100 90 110]  Measurements=None  LoadType=constant Z
  Three-Phase Series RLC Load16 : spsThreePhaseSeriesRLCLoadLib/Three-Phase Series RLC Load  LConnTagsString=A|B|C  Configuration=Y (grounded)  NominalVoltage=1  Vabc=[1e3 1e3 1e3]  Vabcp=[1e3 1e3 1e3]  NominalFrequency=50  UnbalancedPower=off  ActivePower=0.175  InductivePower=0.112  CapacitivePower=0  Pabc=[10e3 9e3 11e3]  QLabc=[100 90 110]  QCabc=[100 90 110]  Pabcp=[10e3 9e3 11e3]  QLabcp=[100 90 110]  QCabcp=[100 90 110]  Measurements=None  LoadType=constant Z
  Three-Phase Series RLC Load17 : spsThreePhaseSeriesRLCLoadLib/Three-Phase Series RLC Load  LConnTagsString=A|B|C  Configuration=Y (grounded)  NominalVoltage=1  Vabc=[1e3 1e3 1e3]  Vabcp=[1e3 1e3 1e3]  NominalFrequency=50  UnbalancedPower=off  ActivePower=0.032  InductivePower=0.016  CapacitivePower=0  Pabc=[10e3 9e3 11e3]  QLabc=[100 90 110]  QCabc=[100 90 110]  Pabcp=[10e3 9e3 11e3]  QLabcp=[100 90 110]  QCabcp=[100 90 110]  Measurements=None  LoadType=constant Z
  Three-Phase Series RLC Load18 : spsThreePhaseSeriesRLCLoadLib/Three-Phase Series RLC Load  LConnTagsString=A|B|C  Configuration=Y (grounded)  NominalVoltage=1  Vabc=[1e3 1e3 1e3]  Vabcp=[1e3 1e3 1e3]  NominalFrequency=50  UnbalancedPower=off  ActivePower=0.087  InductivePower=0.067  CapacitivePower=0  Pabc=[10e3 9e3 11e3]  QLabc=[100 90 110]  QCabc=[100 90 110]  Pabcp=[10e3 9e3 11e3]  QLabcp=[100 90 110]  QCabcp=[100 90 110]  Measurements=None  LoadType=constant Z
  Three-Phase Series RLC Load19 : spsThreePhaseSeriesRLCLoadLib/Three-Phase Series RLC Load  LConnTagsString=A|B|C  Configuration=Y (grounded)  NominalVoltage=1  Vabc=[1e3 1e3 1e3]  Vabcp=[1e3 1e3 1e3]  NominalFrequency=50  UnbalancedPower=off  ActivePower=0.035  InductivePower=0.023  CapacitivePower=0  Pabc=[10e3 9e3 11e3]  QLabc=[100 90 110]  QCabc=[100 90 110]  Pabcp=[10e3 9e3 11e3]  QLabcp=[100 90 110]  QCabcp=[100 90 110]  Measurements=None  LoadType=constant Z
  Three-Phase Series RLC Load2 : spsThreePhaseSeriesRLCLoadLib/Three-Phase Series RLC Load  LConnTagsString=A|B|C  Configuration=Y (grounded)  NominalVoltage=1  Vabc=[1e3 1e3 1e3]  Vabcp=[1e3 1e3 1e3]  NominalFrequency=50  UnbalancedPower=off  ActivePower=0.076  InductivePower=0.016  CapacitivePower=0  Pabc=[10e3 9e3 11e3]  QLabc=[100 90 110]  QCabc=[100 90 110]  Pabcp=[10e3 9e3 11e3]  QLabcp=[100 90 110]  QCabcp=[100 90 110]  Measurements=None  LoadType=constant Z
  Three-Phase Series RLC Load21 : spsThreePhaseSeriesRLCLoadLib/Three-Phase Series RLC Load  LConnTagsString=A|B|C  Configuration=Y (grounded)  NominalVoltage=1  Vabc=[1e3 1e3 1e3]  Vabcp=[1e3 1e3 1e3]  NominalFrequency=50  UnbalancedPower=off  ActivePower=0.024  InductivePower=0.009  CapacitivePower=0  Pabc=[10e3 9e3 11e3]  QLabc=[100 90 110]  QCabc=[100 90 110]  Pabcp=[10e3 9e3 11e3]  QLabcp=[100 90 110]  QCabcp=[100 90 110]  Measurements=None  LoadType=constant Z
  Three-Phase Series RLC Load22 : spsThreePhaseSeriesRLCLoadLib/Three-Phase Series RLC Load  LConnTagsString=A|B|C  Configuration=Y (grounded)  NominalVoltage=1  Vabc=[1e3 1e3 1e3]  Vabcp=[1e3 1e3 1e3]  NominalFrequency=50  UnbalancedPower=off  ActivePower=0.106  InductivePower=0.019  CapacitivePower=0  Pabc=[10e3 9e3 11e3]  QLabc=[100 90 110]  QCabc=[100 90 110]  Pabcp=[10e3 9e3 11e3]  QLabcp=[100 90 110]  QCabcp=[100 90 110]  Measurements=None  LoadType=constant Z
  Three-Phase Series RLC Load3 : spsThreePhaseSeriesRLCLoadLib/Three-Phase Series RLC Load  LConnTagsString=A|B|C  Configuration=Y (grounded)  NominalVoltage=1  Vabc=[1e3 1e3 1e3]  Vabcp=[1e3 1e3 1e3]  NominalFrequency=50  UnbalancedPower=off  ActivePower=0.942  InductivePower=0.19  CapacitivePower=0  Pabc=[10e3 9e3 11e3]  QLabc=[100 90 110]  QCabc=[100 90 110]  Pabcp=[10e3 9e3 11e3]  QLabcp=[100 90 110]  QCabcp=[100 90 110]  Measurements=None  LoadType=constant Z
  Three-Phase Series RLC Load5 : spsThreePhaseSeriesRLCLoadLib/Three-Phase Series RLC Load  LConnTagsString=A|B|C  Configuration=Y (grounded)  NominalVoltage=1  Vabc=[1e3 1e3 1e3]  Vabcp=[1e3 1e3 1e3]  NominalFrequency=50  UnbalancedPower=off  ActivePower=0.228  InductivePower=0.109  CapacitivePower=0  Pabc=[10e3 9e3 11e3]  QLabc=[100 90 110]  QCabc=[100 90 110]  Pabcp=[10e3 9e3 11e3]  QLabcp=[100 90 110]  QCabcp=[100 90 110]  Measurements=None  LoadType=constant Z
  Three-Phase Series RLC Load6 : spsThreePhaseSeriesRLCLoadLib/Three-Phase Series RLC Load  LConnTagsString=A|B|C  Configuration=Y (grounded)  NominalVoltage=1  Vabc=[1e3 1e3 1e3]  Vabcp=[1e3 1e3 1e3]  NominalFrequency=50  UnbalancedPower=off  ActivePower=0.035  InductivePower=0.018  CapacitivePower=0  Pabc=[10e3 9e3 11e3]  QLabc=[100 90 110]  QCabc=[100 90 110]  Pabcp=[10e3 9e3 11e3]  QLabcp=[100 90 110]  QCabcp=[100 90 110]  Measurements=None  LoadType=constant Z
  Three-Phase Series RLC Load7 : spsThreePhaseSeriesRLCLoadLib/Three-Phase Series RLC Load  LConnTagsString=A|B|C  Configuration=Y (grounded)  NominalVoltage=1  Vabc=[1e3 1e3 1e3]  Vabcp=[1e3 1e3 1e3]  NominalFrequency=50  UnbalancedPower=off  ActivePower=0.058  InductivePower=0.02  CapacitivePower=0  Pabc=[10e3 9e3 11e3]  QLabc=[100 90 110]  QCabc=[100 90 110]  Pabcp=[10e3 9e3 11e3]  QLabcp=[100 90 110]  QCabcp=[100 90 110]  Measurements=None  LoadType=constant Z
  Three-Phase Series RLC Load8 : spsThreePhaseSeriesRLCLoadLib/Three-Phase Series RLC Load  LConnTagsString=A|B|C  Configuration=Y (grounded)  NominalVoltage=1  Vabc=[1e3 1e3 1e3]  Vabcp=[1e3 1e3 1e3]  NominalFrequency=50  UnbalancedPower=off  ActivePower=0.09  InductivePower=0.058  CapacitivePower=0  Pabc=[10e3 9e3 11e3]  QLabc=[100 90 110]  QCabc=[100 90 110]  Pabcp=[10e3 9e3 11e3]  QLabcp=[100 90 110]  QCabcp=[100 90 110]  Measurements=None  LoadType=constant Z
  Three-Phase Series RLC Load9 : spsThreePhaseSeriesRLCLoadLib/Three-Phase Series RLC Load  LConnTagsString=A|B|C  Configuration=Y (grounded)  NominalVoltage=1  Vabc=[1e3 1e3 1e3]  Vabcp=[1e3 1e3 1e3]  NominalFrequency=50  UnbalancedPower=off  ActivePower=0.112  InductivePower=0.075  CapacitivePower=0  Pabc=[10e3 9e3 11e3]  QLabc=[100 90 110]  QCabc=[100 90 110]  Pabcp=[10e3 9e3 11e3]  QLabcp=[100 90 110]  QCabcp=[100 90 110]  Measurements=None  LoadType=constant Z
  Three-Phase Transformer (Two Windings) : spsThreePhaseTransformerTwoWindingsLib/Three-Phase Transformer (Two Windings)  Winding1Connection=Yg  Winding2Connection=Yg  CoreType=Three single-phase transformers  SetSaturation=off  Hysteresis=off  DataFile='hysteresis'  SetInitialFlux=off  Measurements=None  UNITS=pu  NominalPower=[ 1 , 50 ]  Winding1=[1.06 , 0.002 , 0.08 ]  Winding2=[ 1.06 , 0.002 , 0.08 ]  Rm=500  Lm=500  L0=0.5  Saturation=[ 0,0 ; 0.0024,1.2 ; 1.0,1.52 ]  InitialFluxes=[ 0.8 , -0.8 , 0.7 ]  BreakLoop=off  DiscreteSolver=Trapezoidal iterative  DataType=off  TransfoNumber=1
  Three-Phase Transformer (Two Windings)1 : spsThreePhaseTransformerTwoWindingsLib/Three-Phase Transformer (Two Windings)  Winding1Connection=Yg  Winding2Connection=Yg  CoreType=Three single-phase transformers  SetSaturation=off  Hysteresis=off  DataFile='hysteresis'  SetInitialFlux=off  Measurements=None  UNITS=pu  NominalPower=[1 , 50 ]  Winding1=[ 1.045 , 0.002 , 0.08 ]  Winding2=[ 1.045 , 0.002 , 0.08 ]  Rm=500  Lm=500  L0=0.5  Saturation=[ 0,0 ; 0.0024,1.2 ; 1.0,1.52 ]  InitialFluxes=[ 0.8 , -0.8 , 0.7 ]  BreakLoop=off  DiscreteSolver=Trapezoidal iterative  DataType=off  TransfoNumber=1
  Three-Phase Transformer (Two Windings)2 : spsThreePhaseTransformerTwoWindingsLib/Three-Phase Transformer (Two Windings)  Winding1Connection=Yg  Winding2Connection=Yg  CoreType=Three single-phase transformers  SetSaturation=off  Hysteresis=off  DataFile='hysteresis'  SetInitialFlux=off  Measurements=None  UNITS=pu  NominalPower=[ 1 , 50 ]  Winding1=[ 1.010 , 0.002 , 0.08 ]  Winding2=[ 1.010 , 0.002 , 0.08 ]  Rm=500  Lm=500  L0=0.5  Saturation=[ 0,0 ; 0.0024,1.2 ; 1.0,1.52 ]  InitialFluxes=[ 0.8 , -0.8 , 0.7 ]  BreakLoop=off  DiscreteSolver=Trapezoidal iterative  DataType=off  TransfoNumber=1
  Three-Phase Transformer (Two Windings)3 : spsThreePhaseTransformerTwoWindingsLib/Three-Phase Transformer (Two Windings)  Winding1Connection=Yg  Winding2Connection=Yg  CoreType=Three single-phase transformers  SetSaturation=off  Hysteresis=off  DataFile='hysteresis'  SetInitialFlux=off  Measurements=None  UNITS=pu  NominalPower=[ 250e6 , 60 ]  Winding1=[ 735e3 , 0.002 , 0.08 ]  Winding2=[ 315e3 , 0.002 , 0.08 ]  Rm=500  Lm=500  L0=0.5  Saturation=[ 0,0 ; 0.0024,1.2 ; 1.0,1.52 ]  InitialFluxes=[ 0.8 , -0.8 , 0.7 ]  BreakLoop=off  DiscreteSolver=Trapezoidal iterative  DataType=off  TransfoNumber=1
  Three-Phase Transformer (Two Windings)4 : spsThreePhaseTransformerTwoWindingsLib/Three-Phase Transformer (Two Windings)  Winding1Connection=Yg  Winding2Connection=Yg  CoreType=Three single-phase transformers  SetSaturation=off  Hysteresis=off  DataFile='hysteresis'  SetInitialFlux=off  Measurements=None  UNITS=pu  NominalPower=[ 1 , 50 ]  Winding1=[ 1.082 , 0.002 , 0.08 ]  Winding2=[ 1.082 , 0.002 , 0.08 ]  Rm=500  Lm=500  L0=0.5  Saturation=[ 0,0 ; 0.0024,1.2 ; 1.0,1.52 ]  InitialFluxes=[ 0.8 , -0.8 , 0.7 ]  BreakLoop=off  DiscreteSolver=Trapezoidal iterative  DataType=off  TransfoNumber=1
  Three-Phase Transformer (Two Windings)5 : spsThreePhaseTransformerTwoWindingsLib/Three-Phase Transformer (Two Windings)  Winding1Connection=Yg  Winding2Connection=Yg  CoreType=Three single-phase transformers  SetSaturation=off  Hysteresis=off  DataFile='hysteresis'  SetInitialFlux=off  Measurements=None  UNITS=pu  NominalPower=[ 1 , 50 ]  Winding1=[ 1.071 , 0.002 , 0.08 ]  Winding2=[ 1.071 , 0.002 , 0.08 ]  Rm=500  Lm=500  L0=0.5  Saturation=[ 0,0 ; 0.0024,1.2 ; 1.0,1.52 ]  InitialFluxes=[ 0.8 , -0.8 , 0.7 ]  BreakLoop=off  DiscreteSolver=Trapezoidal iterative  DataType=off  TransfoNumber=1
  powergui : spspowerguiLib/powergui  Priority=1  SimulationMode=Discrete  SampleTime=50e-6  frequency=60  Iterations=50  frequencyindice=50  Pbase=100e6  ErrMax=1e-4  UnitsV=kV  UnitsW=MW  buscounter=0  FunctionMessages=off  echomessages=off  EnableUseOfTLC=off  CurrentSourceSwitches=off  DisableSnubberDevices=off  DisableRonSwitches=off  DisableVfSwitches=off  DisplayEquations=off  AutomaticDiscreteSolvers=off  SolverType=Tustin/Backward Euler (TBE)  Interpol=off  ExternalGateDelay=off  methode=off  Ts=10  x0status=blocks  SPID=off  SwTol=0  HookPort=off  NonlinearTolerance=1e-4  nMaxIteration=100  ContinueOnMaxIteration=off  RestoreLinks=warning  ResistiveCurrentMeasurement=off  Frange=[0:2:500]  Ylog=off  Xlog=on  ShowGrid=off  save=off  variable=ZData  structure=0  ZoomFFT=off  StartTime=0.0  cycles=1  DisplayStyle=1  fundamental=60  FreqAxis=off  MaxFrequency=1000  frequencyindicesteady=1  RmsSteady=1  display=off
  wires:
  Subsystem/1(Out1) -> Scope2/1
  [Vabc_1] -> Subsystem/1(In1)
  Subsystem/2(Out2) -> Scope2/2
  Subsystem/3(Out3) -> Scope2/3
  Subsystem/4(Out4) -> Scope2/4
  Subsystem/5(Out5) -> Scope2/5
  Subsystem/6(Out6) -> Scope2/6
  Subsystem/7(Out7) -> Scope2/7
  Subsystem/8(Out8) -> Scope2/8
  Subsystem/9(Out9) -> Scope2/9
  Subsystem/10(Out10) -> Scope2/10
  Subsystem/11(Out11) -> Scope2/11
  Subsystem/12(Out12) -> Scope2/12
  Subsystem/13(Out13) -> Scope2/13
  Subsystem/14(Out14) -> Scope2/14
  Subsystem/15(Out15) -> Scope2/15
  Subsystem/16(Out16) -> Scope2/16
  [Vabc_2] -> Subsystem/2(In2)
  [Vabc_3] -> Subsystem/3(In3)
  [Vabc_4] -> Subsystem/4(In4)
  [Vabc_5] -> Subsystem/5(In5)
  [Vabc_6] -> Subsystem/6(In6)
  [Vabc_7] -> Subsystem/7(In7)
  [Vabc_8] -> Subsystem/8(In8)
  [Vabc_9] -> Subsystem/9(In9)
  [Vabc_10] -> Subsystem/10(In10)
  [Vabc_11] -> Subsystem/11(In11)
  [Vabc_12] -> Subsystem/12(In12)
  [Vabc_13] -> Subsystem/13(In13)
  [Vabc_14] -> Subsystem/14(In14)
  [Vabc_15] -> Subsystem/15(In15)
  [Vabc_16] -> Subsystem/16(In16)
  [Vabc_22] -> Subsystem1/6(In6)
  [Vabc_24] -> Subsystem1/8(In8)
  Subsystem1/14(Out14) -> Scope1/14
  [Vabc_21] -> Subsystem1/5(In5)
  Subsystem1/8(Out8) -> Scope1/8
  Subsystem1/6(Out6) -> Scope1/6
  Subsystem1/7(Out7) -> Scope1/7
  Subsystem1/5(Out5) -> Scope1/5
  Subsystem1/11(Out11) -> Scope1/11
  [Vabc_29] -> Subsystem1/13(In13)
  [Vabc_20] -> Subsystem1/4(In4)
  [Vabc_27] -> Subsystem1/11(In11)
  [Vabc_25] -> Subsystem1/9(In9)
  Subsystem1/12(Out12) -> Scope1/12
  Subsystem1/13(Out13) -> Scope1/13
  [Vabc_23] -> Subsystem1/7(In7)
  Subsystem1/3(Out3) -> Scope1/3
  Subsystem1/2(Out2) -> Scope1/2
  [Vabc_18] -> Subsystem1/2(In2)
  [Vabc_28] -> Subsystem1/12(In12)
  Subsystem1/1(Out1) -> Scope1/1
  [Vabc_30] -> Subsystem1/14(In14)
  Subsystem1/9(Out9) -> Scope1/9
  Subsystem1/10(Out10) -> Scope1/10
  [Vabc_19] -> Subsystem1/3(In3)
  [Vabc_26] -> Subsystem1/10(In10)
  Subsystem1/4(Out4) -> Scope1/4
  [Vabc_17] -> Subsystem1/1(In1)
  [Iabc_15] -> Subsystem2/15(In15)
  [Iabc_6] -> Subsystem2/6(In6)
  [Iabc_8] -> Subsystem2/8(In8)
  Subsystem2/14(Out14) -> Scope3/14
  [Iabc_5] -> Subsystem2/5(In5)
  Subsystem2/8(Out8) -> Scope3/8
  Subsystem2/6(Out6) -> Scope3/6
  Subsystem2/7(Out7) -> Scope3/7
  Subsystem2/5(Out5) -> Scope3/5
  Subsystem2/11(Out11) -> Scope3/11
  [Iabc_13] -> Subsystem2/13(In13)
  [Iabc_4] -> Subsystem2/4(In4)
  [Iabc_11] -> Subsystem2/11(In11)
  [Iabc_9] -> Subsystem2/9(In9)
  Subsystem2/12(Out12) -> Scope3/12
  Subsystem2/15(Out15) -> Scope3/15
  [Iabc_16] -> Subsystem2/16(In16)
  Subsystem2/13(Out13) -> Scope3/13
  [Iabc_7] -> Subsystem2/7(In7)
  Subsystem2/3(Out3) -> Scope3/3
  Subsystem2/2(Out2) -> Scope3/2
  [Iabc_2] -> Subsystem2/2(In2)
  [Iabc_12] -> Subsystem2/12(In12)
  Subsystem2/1(Out1) -> Scope3/1
  [Iabc_14] -> Subsystem2/14(In14)
  Subsystem2/9(Out9) -> Scope3/9
  Subsystem2/10(Out10) -> Scope3/10
  [Iabc_3] -> Subsystem2/3(In3)
  [Iabc_10] -> Subsystem2/10(In10)
  Subsystem2/16(Out16) -> Scope3/16
  Subsystem2/4(Out4) -> Scope3/4
  [Iabc_1] -> Subsystem2/1(In1)
  Subsystem3/1(Out1) -> Scope4/1
  Subsystem3/4(Out4) -> Scope4/4
  [Iabc_30] -> Subsystem3/14(In14)
  [Iabc_19] -> Subsystem3/3(In3)
  [Iabc_26] -> Subsystem3/10(In10)
  Subsystem3/9(Out9) -> Scope4/9
  [Iabc_17] -> Subsystem3/1(In1)
  Subsystem3/12(Out12) -> Scope4/12
  Subsystem3/13(Out13) -> Scope4/13
  Subsystem3/3(Out3) -> Scope4/3
  [Iabc_28] -> Subsystem3/12(In12)
  Subsystem3/2(Out2) -> Scope4/2
  [Iabc_18] -> Subsystem3/2(In2)
  [Iabc_20] -> Subsystem3/4(In4)
  Subsystem3/8(Out8) -> Scope4/8
  [Iabc_29] -> Subsystem3/13(In13)
  Subsystem3/11(Out11) -> Scope4/11
  [Iabc_23] -> Subsystem3/7(In7)
  Subsystem3/7(Out7) -> Scope4/7
  Subsystem3/6(Out6) -> Scope4/6
  Subsystem3/10(Out10) -> Scope4/10
  [Iabc_21] -> Subsystem3/5(In5)
  Subsystem3/5(Out5) -> Scope4/5
  [Iabc_25] -> Subsystem3/9(In9)
  Subsystem3/14(Out14) -> Scope4/14
  [Iabc_27] -> Subsystem3/11(In11)
  [Iabc_24] -> Subsystem3/8(In8)
  [Iabc_22] -> Subsystem3/6(In6)
  connections:
  Gen1/RConn3 -- Three-Phase Transformer (Two Windings)/LConn3
  Gen1/RConn2 -- Three-Phase Transformer (Two Windings)/LConn2
  Gen1/RConn1 -- Three-Phase Transformer (Two Windings)/LConn1
  Gen2/RConn1 -- Three-Phase Transformer (Two Windings)1/LConn1
  Gen2/RConn2 -- Three-Phase Transformer (Two Windings)1/LConn2
  Gen2/RConn3 -- Three-Phase Transformer (Two Windings)1/LConn3
  Gen3/RConn1 -- Three-Phase Transformer (Two Windings)2/LConn1
  Gen3/RConn2 -- Three-Phase Transformer (Two Windings)2/LConn2
  Gen3/RConn3 -- Three-Phase Transformer (Two Windings)2/LConn3
  Gen4/RConn1 -- Three-Phase Transformer (Two Windings)3/LConn1
  Gen4/RConn2 -- Three-Phase Transformer (Two Windings)3/LConn2
  Gen4/RConn3 -- Three-Phase Transformer (Two Windings)3/LConn3
  Gen5/RConn1 -- Three-Phase Transformer (Two Windings)4/LConn1
  Gen5/RConn2 -- Three-Phase Transformer (Two Windings)4/LConn2
  Gen5/RConn3 -- Three-Phase Transformer (Two Windings)4/LConn3
  Gen6/RConn1 -- Three-Phase Transformer (Two Windings)5/LConn1
  Gen6/RConn2 -- Three-Phase Transformer (Two Windings)5/LConn2
  Gen6/RConn3 -- Three-Phase Transformer (Two Windings)5/LConn3
  Three-Phase Series RLC Load1/LConn1 -- Bus 3/RConn1
  Three-Phase Series RLC Load1/LConn2 -- Bus 3/RConn2
  Three-Phase Series RLC Load1/LConn3 -- Bus 3/RConn3
  Three-Phase Series RLC Load2/LConn2 -- Bus 4/RConn2
  Three-Phase Series RLC Load2/LConn3 -- Bus 4/RConn3
  Three-Phase Series RLC Load2/LConn1 -- Bus 4/RConn1
  Three-Phase Series RLC Load5/LConn2 -- Bus 7/RConn2
  Three-Phase Series RLC Load5/LConn3 -- Bus 7/RConn3
  Three-Phase Series RLC Load5/LConn1 -- Bus 7/RConn1
  Three-Phase Series RLC Load7/LConn3 -- Bus 10/RConn3
  Three-Phase Series RLC Load7/LConn2 -- Bus 10/RConn2
  Three-Phase Series RLC Load7/LConn1 -- Bus 10/RConn1
  Three-Phase Series RLC Load9/LConn3 -- Bus 12/RConn3
  Three-Phase Series RLC Load9/LConn2 -- Bus 12/RConn2
  Three-Phase Series RLC Load9/LConn1 -- Bus 12/RConn1
  Three-Phase Series RLC Load10/LConn3 -- Bus 14/RConn3
  Three-Phase Series RLC Load10/LConn2 -- Bus 14/RConn2
  Three-Phase Series RLC Load10/LConn1 -- Bus 14/RConn1
  Three-Phase Series RLC Load11/LConn3 -- Bus 15/RConn3
  Three-Phase Series RLC Load11/LConn2 -- Bus 15/RConn2
  Three-Phase Series RLC Load11/LConn1 -- Bus 15/RConn1
  Three-Phase Transformer (Two Windings)/RConn1 -- Bus 1/RConn1
  Three-Phase Transformer (Two Windings)/RConn2 -- Bus 1/RConn2
  Three-Phase Transformer (Two Windings)/RConn3 -- Bus 1/RConn3
  Three-Phase Transformer (Two Windings)1/RConn1 -- Three-Phase Series RLC Load/LConn1 -- Bus 2/RConn1
  Three-Phase Transformer (Two Windings)1/RConn2 -- Three-Phase Series RLC Load/LConn2 -- Bus 2/RConn2
  Three-Phase Transformer (Two Windings)1/RConn3 -- Three-Phase Series RLC Load/LConn3 -- Bus 2/RConn3
  Three-Phase Transformer (Two Windings)2/RConn1 -- Three-Phase Series RLC Load3/LConn1 -- Bus 5/RConn1
  Three-Phase Transformer (Two Windings)2/RConn2 -- Three-Phase Series RLC Load3/LConn2 -- Bus 5/RConn2
  Three-Phase Transformer (Two Windings)2/RConn3 -- Three-Phase Series RLC Load3/LConn3 -- Bus 5/RConn3
  Three-Phase Transformer (Two Windings)3/RConn1 -- Three-Phase Series RLC Load12/LConn1 -- Bus 8/RConn1
  Three-Phase Transformer (Two Windings)3/RConn2 -- Three-Phase Series RLC Load12/LConn2 -- Bus 8/RConn2
  Three-Phase Transformer (Two Windings)3/RConn3 -- Three-Phase Series RLC Load12/LConn3 -- Bus 8/RConn3
  Three-Phase Transformer (Two Windings)4/RConn1 -- Bus 11/RConn1
  Three-Phase Transformer (Two Windings)4/RConn2 -- Bus 11/RConn2
  Three-Phase Transformer (Two Windings)4/RConn3 -- Bus 11/RConn3
  Three-Phase Transformer (Two Windings)5/RConn1 -- Bus 13/RConn1
  Three-Phase Transformer (Two Windings)5/RConn2 -- Bus 13/RConn2
  Three-Phase Transformer (Two Windings)5/RConn3 -- Bus 13/RConn3
  Three-Phase Series RLC Branch/LConn1 -- Three-Phase Series RLC Branch1/LConn1 -- Bus 1/LConn1
  Three-Phase Series RLC Branch/LConn2 -- Three-Phase Series RLC Branch1/LConn2 -- Bus 1/LConn2
  Three-Phase Series RLC Branch/LConn3 -- Three-Phase Series RLC Branch1/LConn3 -- Bus 1/LConn3
  Three-Phase Series RLC Branch/RConn1 -- Three-Phase Series RLC Branch5/LConn1 -- Three-Phase Series RLC Branch4/LConn1 -- Three-Phase Series RLC Branch3/LConn1 -- Bus 2/LConn1
  Three-Phase Series RLC Branch/RConn2 -- Three-Phase Series RLC Branch5/LConn2 -- Three-Phase Series RLC Branch4/LConn2 -- Three-Phase Series RLC Branch3/LConn2 -- Bus 2/LConn2
  Three-Phase Series RLC Branch/RConn3 -- Three-Phase Series RLC Branch5/LConn3 -- Three-Phase Series RLC Branch4/LConn3 -- Three-Phase Series RLC Branch3/LConn3 -- Bus 2/LConn3
  Three-Phase Series RLC Branch1/RConn1 -- Three-Phase Series RLC Branch2/LConn1 -- Bus 3/LConn1
  Three-Phase Series RLC Branch1/RConn2 -- Three-Phase Series RLC Branch2/LConn2 -- Bus 3/LConn2
  Three-Phase Series RLC Branch1/RConn3 -- Three-Phase Series RLC Branch2/LConn3 -- Bus 3/LConn3
  Three-Phase Series RLC Branch2/RConn1 -- Three-Phase Series RLC Branch6/LConn1 -- Bus 4/LConn1 -- Three-Phase Series RLC Branch17/LConn1 -- Three-Phase Series RLC Branch3/RConn1
  Three-Phase Series RLC Branch2/RConn2 -- Three-Phase Series RLC Branch6/LConn2 -- Bus 4/LConn2 -- Three-Phase Series RLC Branch17/LConn2 -- Three-Phase Series RLC Branch3/RConn2
  Three-Phase Series RLC Branch2/RConn3 -- Three-Phase Series RLC Branch6/LConn3 -- Bus 4/LConn3 -- Three-Phase Series RLC Branch17/LConn3 -- Three-Phase Series RLC Branch3/RConn3
  Bus 5/LConn1 -- Three-Phase Series RLC Branch8/LConn1 -- Three-Phase Series RLC Branch4/RConn1 -- 3-Phase Fault/LConn1
  Bus 5/LConn2 -- 3-Phase Fault/LConn2 -- Three-Phase Series RLC Branch8/LConn2 -- Three-Phase Series RLC Branch4/RConn2
  Bus 5/LConn3 -- 3-Phase Fault/LConn3 -- Three-Phase Series RLC Branch8/LConn3 -- Three-Phase Series RLC Branch4/RConn3
  Bus 6/LConn1 -- Three-Phase Series RLC Branch6/RConn1 -- Three-Phase Series RLC Branch9/LConn1 -- Three-Phase Series RLC Branch10/LConn1 -- Three-Phase Series RLC Branch5/RConn1 -- Three-Phase Series RLC Branch37/LConn1 -- Three-Phase Series RLC Branch12/LConn1
  Bus 6/LConn2 -- Three-Phase Series RLC Branch6/RConn2 -- Three-Phase Series RLC Branch9/LConn2 -- Three-Phase Series RLC Branch10/LConn2 -- Three-Phase Series RLC Branch12/LConn2 -- Three-Phase Series RLC Branch5/RConn2 -- Three-Phase Series RLC Branch37/LConn2
  Bus 6/LConn3 -- Three-Phase Series RLC Branch6/RConn3 -- Three-Phase Series RLC Branch9/LConn3 -- Three-Phase Series RLC Branch10/LConn3 -- Three-Phase Series RLC Branch12/LConn3 -- Three-Phase Series RLC Branch5/RConn3 -- Three-Phase Series RLC Branch37/LConn3
  Three-Phase Series RLC Branch7/RConn1 -- Bus 7/LConn1 -- Three-Phase Series RLC Branch8/RConn1
  Three-Phase Series RLC Branch7/RConn2 -- Three-Phase Series RLC Branch8/RConn2 -- Bus 7/LConn2
  Three-Phase Series RLC Branch7/RConn3 -- Three-Phase Series RLC Branch8/RConn3 -- Bus 7/LConn3
  Three-Phase Series RLC Branch9/RConn1 -- Three-Phase Series RLC Branch38/LConn1 -- Bus 8/LConn1
  Three-Phase Series RLC Branch9/RConn2 -- Bus 8/LConn2 -- Three-Phase Series RLC Branch38/LConn2
  Three-Phase Series RLC Branch9/RConn3 -- Three-Phase Series RLC Branch38/LConn3 -- Bus 8/LConn3
  Three-Phase Series RLC Branch10/RConn1 -- Three-Phase Series RLC Branch13/LConn1 -- Bus 9/LConn1
  Three-Phase Series RLC Branch10/RConn2 -- Three-Phase Series RLC Branch13/LConn2 -- Bus 9/LConn2
  Three-Phase Series RLC Branch10/RConn3 -- Three-Phase Series RLC Branch13/LConn3 -- Bus 9/LConn3
  Three-Phase Series RLC Branch11/LConn1 -- Bus 9/RConn1
  Three-Phase Series RLC Branch11/LConn2 -- Bus 9/RConn2
  Three-Phase Series RLC Branch11/LConn3 -- Bus 9/RConn3
  Three-Phase Series RLC Branch11/RConn1 -- Three-Phase Series RLC Branch12/RConn1 -- Three-Phase Series RLC Branch25/LConn1 -- Three-Phase Series RLC Branch27/RConn1 -- Three-Phase Series RLC Branch24/LConn1 -- Three-Phase Series RLC Branch20/LConn1 -- Bus 10/LConn1
  Three-Phase Series RLC Branch11/RConn2 -- Three-Phase Series RLC Branch12/RConn2 -- Three-Phase Series RLC Branch25/LConn2 -- Three-Phase Series RLC Branch27/RConn2 -- Three-Phase Series RLC Branch24/LConn2 -- Three-Phase Series RLC Branch20/LConn2 -- Bus 10/LConn2
  Three-Phase Series RLC Branch11/RConn3 -- Three-Phase Series RLC Branch12/RConn3 -- Three-Phase Series RLC Branch25/LConn3 -- Three-Phase Series RLC Branch27/RConn3 -- Three-Phase Series RLC Branch24/LConn3 -- Three-Phase Series RLC Branch20/LConn3 -- Bus 10/LConn3
  Three-Phase Series RLC Branch13/RConn1 -- 3-Phase Fault1/LConn1 -- Bus 11/LConn1
  Three-Phase Series RLC Branch13/RConn2 -- 3-Phase Fault1/LConn2 -- Bus 11/LConn2
  Three-Phase Series RLC Branch13/RConn3 -- 3-Phase Fault1/LConn3 -- Bus 11/LConn3
  Three-Phase Series RLC Branch14/LConn1 -- Three-Phase Series RLC Branch39/LConn1 -- Three-Phase Series RLC Branch18/LConn1 -- Three-Phase Series RLC Branch15/LConn1 -- Bus 12/LConn1
  Three-Phase Series RLC Branch14/LConn2 -- Three-Phase Series RLC Branch39/LConn2 -- Three-Phase Series RLC Branch18/LConn2 -- Three-Phase Series RLC Branch15/LConn2 -- Bus 12/LConn2
  Three-Phase Series RLC Branch14/LConn3 -- Three-Phase Series RLC Branch39/LConn3 -- Three-Phase Series RLC Branch18/LConn3 -- Three-Phase Series RLC Branch15/LConn3 -- Bus 12/LConn3
  Three-Phase Series RLC Branch14/RConn1 -- Bus 13/LConn1
  Three-Phase Series RLC Branch14/RConn2 -- Bus 13/LConn2
  Three-Phase Series RLC Branch14/RConn3 -- Bus 13/LConn3
  Three-Phase Series RLC Branch15/RConn1 -- Three-Phase Series RLC Branch16/LConn1 -- Bus 14/LConn1
  Three-Phase Series RLC Branch15/RConn2 -- Three-Phase Series RLC Branch16/LConn2 -- Bus 14/LConn2
  Three-Phase Series RLC Branch15/RConn3 -- Three-Phase Series RLC Branch16/LConn3 -- Bus 14/LConn3
  Three-Phase Series RLC Branch16/RConn1 -- Three-Phase Series RLC Branch39/RConn1 -- Three-Phase Series RLC Branch21/LConn1 -- Three-Phase Series RLC Branch28/LConn1 -- Three-Phase Series RLC Branch17/RConn1 -- Bus 15/LConn1
  Three-Phase Series RLC Branch16/RConn2 -- Three-Phase Series RLC Branch39/RConn2 -- Three-Phase Series RLC Branch21/LConn2 -- Three-Phase Series RLC Branch28/LConn2 -- Three-Phase Series RLC Branch17/RConn2 -- Bus 15/LConn2
  Three-Phase Series RLC Branch16/RConn3 -- Three-Phase Series RLC Branch39/RConn3 -- Three-Phase Series RLC Branch21/LConn3 -- Three-Phase Series RLC Branch28/LConn3 -- Three-Phase Series RLC Branch17/RConn3 -- Bus 15/LConn3
  Three-Phase Series RLC Load6/LConn1 -- Bus 16/LConn1
  Three-Phase Series RLC Load6/LConn2 -- Bus 16/LConn2
  Three-Phase Series RLC Load6/LConn3 -- Bus 16/LConn3
  Three-Phase Series RLC Load8/LConn1 -- Bus 17/LConn1
  Three-Phase Series RLC Load8/LConn2 -- Bus 17/LConn2
  Three-Phase Series RLC Load8/LConn3 -- Bus 17/LConn3
  Three-Phase Series RLC Load13/LConn1 -- Bus 18/LConn1
  Three-Phase Series RLC Load13/LConn2 -- Bus 18/LConn2
  Three-Phase Series RLC Load13/LConn3 -- Bus 18/LConn3
  Three-Phase Series RLC Load14/LConn1 -- Bus 19/LConn1
  Three-Phase Series RLC Load14/LConn2 -- Bus 19/LConn2
  Three-Phase Series RLC Load14/LConn3 -- Bus 19/LConn3
  Three-Phase Series RLC Load15/LConn1 -- Bus 20/LConn1
  Three-Phase Series RLC Load15/LConn2 -- Bus 20/LConn2
  Three-Phase Series RLC Load15/LConn3 -- Bus 20/LConn3
  Three-Phase Series RLC Load17/LConn1 -- Bus 23/LConn1
  Three-Phase Series RLC Load17/LConn2 -- Bus 23/LConn2
  Three-Phase Series RLC Load17/LConn3 -- Bus 23/LConn3
  Three-Phase Series RLC Load18/LConn1 -- Bus 24/LConn1
  Three-Phase Series RLC Load18/LConn2 -- Bus 24/LConn2
  Three-Phase Series RLC Load18/LConn3 -- Bus 24/LConn3
  Three-Phase Series RLC Load19/LConn1 -- Bus 26/LConn1
  Three-Phase Series RLC Load19/LConn2 -- Bus 26/LConn2
  Three-Phase Series RLC Load19/LConn3 -- Bus 26/LConn3
  Three-Phase Series RLC Load21/LConn1 -- Bus 29/LConn1
  Three-Phase Series RLC Load21/LConn2 -- Bus 29/LConn2
  Three-Phase Series RLC Load21/LConn3 -- Bus 29/LConn3
  Three-Phase Series RLC Load22/LConn1 -- Bus 30/LConn1
  Three-Phase Series RLC Load22/LConn2 -- Bus 30/LConn2
  Three-Phase Series RLC Load22/LConn3 -- Bus 30/LConn3
  Three-Phase Series RLC Branch18/RConn1 -- Three-Phase Series RLC Branch19/LConn1 -- Three-Phase Series RLC Branch19/LConn2 -- Three-Phase Series RLC Branch19/LConn3 -- Bus 16/RConn1
  Three-Phase Series RLC Branch18/RConn2 -- Bus 16/RConn2
  Three-Phase Series RLC Branch18/RConn3 -- Bus 16/RConn3
  Three-Phase Series RLC Branch19/RConn1 -- Three-Phase Series RLC Branch20/RConn1 -- Bus 17/RConn1
  Three-Phase Series RLC Branch19/RConn2 -- Three-Phase Series RLC Branch20/RConn2 -- Bus 17/RConn2
  Three-Phase Series RLC Branch19/RConn3 -- Three-Phase Series RLC Branch20/RConn3 -- Bus 17/RConn3
  Three-Phase Series RLC Branch21/RConn1 -- Bus 18/RConn1 -- Three-Phase Series RLC Branch22/LConn1
  Three-Phase Series RLC Branch21/RConn2 -- Bus 18/RConn2 -- Three-Phase Series RLC Branch22/LConn2
  Three-Phase Series RLC Branch21/RConn3 -- Bus 18/RConn3 -- Three-Phase Series RLC Branch22/LConn3
  Three-Phase Series RLC Branch22/RConn1 -- Bus 19/RConn1 -- Three-Phase Series RLC Branch23/LConn1
  Three-Phase Series RLC Branch22/RConn2 -- Three-Phase Series RLC Branch23/LConn2 -- Bus 19/RConn2
  Three-Phase Series RLC Branch22/RConn3 -- Bus 19/RConn3 -- Three-Phase Series RLC Branch23/LConn3
  Three-Phase Series RLC Branch23/RConn1 -- Three-Phase Series RLC Branch24/RConn1 -- Bus 20/RConn1
  Three-Phase Series RLC Branch23/RConn2 -- Three-Phase Series RLC Branch24/RConn2 -- Bus 20/RConn2
  Three-Phase Series RLC Branch23/RConn3 -- Three-Phase Series RLC Branch24/RConn3 -- Bus 20/RConn3
  Three-Phase Series RLC Load16/LConn3 -- Bus 21/LConn3
  Three-Phase Series RLC Load16/LConn2 -- Bus 21/LConn2
  Three-Phase Series RLC Load16/LConn1 -- Bus 21/LConn1
  Three-Phase Series RLC Branch25/RConn1 -- Bus 21/RConn1 -- Three-Phase Series RLC Branch26/LConn1
  Three-Phase Series RLC Branch25/RConn2 -- Bus 21/RConn2 -- Three-Phase Series RLC Branch26/LConn2
  Three-Phase Series RLC Branch25/RConn3 -- Bus 21/RConn3 -- Three-Phase Series RLC Branch26/LConn3
  Three-Phase Series RLC Branch26/RConn1 -- Bus 22/RConn1 -- Three-Phase Series RLC Branch29/LConn1
  Three-Phase Series RLC Branch26/RConn2 -- Three-Phase Series RLC Branch29/LConn2 -- Bus 22/RConn2
  Three-Phase Series RLC Branch26/RConn3 -- Bus 22/RConn3 -- Three-Phase Series RLC Branch29/LConn3
  Three-Phase Series RLC Branch28/RConn1 -- Three-Phase Series RLC Branch30/LConn1 -- Bus 23/RConn1
  Three-Phase Series RLC Branch28/RConn2 -- Three-Phase Series RLC Branch30/LConn2 -- Bus 23/RConn2
  Three-Phase Series RLC Branch28/RConn3 -- Three-Phase Series RLC Branch30/LConn3 -- Bus 23/RConn3
  Three-Phase Series RLC Branch29/RConn1 -- Three-Phase Series RLC Branch31/LConn1 -- Three-Phase Series RLC Branch30/RConn1 -- Bus 24/RConn1
  Three-Phase Series RLC Branch29/RConn2 -- Three-Phase Series RLC Branch30/RConn2 -- Bus 24/RConn2 -- Three-Phase Series RLC Branch31/LConn2
  Three-Phase Series RLC Branch29/RConn3 -- Three-Phase Series RLC Branch31/LConn3 -- Three-Phase Series RLC Branch30/RConn3 -- Bus 24/RConn3
  Three-Phase Series RLC Branch31/RConn1 -- Bus 25/RConn1
  Three-Phase Series RLC Branch31/RConn2 -- Bus 25/RConn2
  Three-Phase Series RLC Branch31/RConn3 -- Bus 25/RConn3
  Three-Phase Series RLC Branch32/LConn1 -- Three-Phase Series RLC Branch33/LConn1 -- Bus 25/LConn1
  Bus 25/LConn2 -- Three-Phase Series RLC Branch33/LConn2 -- Three-Phase Series RLC Branch32/LConn2
  Three-Phase Series RLC Branch32/LConn3 -- Three-Phase Series RLC Branch33/LConn3 -- Bus 25/LConn3
  Three-Phase Series RLC Branch32/RConn1 -- Bus 26/RConn1
  Three-Phase Series RLC Branch32/RConn2 -- Bus 26/RConn2
  Three-Phase Series RLC Branch32/RConn3 -- Bus 26/RConn3
  Three-Phase Series RLC Branch35/LConn1 -- Three-Phase Series RLC Branch34/LConn1 -- Three-Phase Series RLC Branch36/RConn1 -- Bus 27/RConn1
  Three-Phase Series RLC Branch35/LConn2 -- Three-Phase Series RLC Branch34/LConn2 -- Three-Phase Series RLC Branch36/RConn2 -- Bus 27/RConn2
  Three-Phase Series RLC Branch35/LConn3 -- Three-Phase Series RLC Branch34/LConn3 -- Three-Phase Series RLC Branch36/RConn3 -- Bus 27/RConn3
  Three-Phase Series RLC Branch34/RConn1 -- Three-Phase Series RLC Branch40/LConn1 -- Bus 29/RConn1
  Three-Phase Series RLC Branch34/RConn2 -- Three-Phase Series RLC Branch40/LConn2 -- Bus 29/RConn2
  Three-Phase Series RLC Branch34/RConn3 -- Three-Phase Series RLC Branch40/LConn3 -- Bus 29/RConn3
  Three-Phase Series RLC Branch35/RConn1 -- Three-Phase Series RLC Branch40/RConn1 -- Bus 30/RConn1
  Three-Phase Series RLC Branch35/RConn2 -- Three-Phase Series RLC Branch40/RConn2 -- Bus 30/RConn2
  Three-Phase Series RLC Branch35/RConn3 -- Three-Phase Series RLC Branch40/RConn3 -- Bus 30/RConn3
  Bus 28/LConn1 -- Three-Phase Series RLC Branch36/LConn1
  Bus 28/LConn2 -- Three-Phase Series RLC Branch36/LConn2
  Bus 28/LConn3 -- Three-Phase Series RLC Branch36/LConn3
  Bus 28/RConn1 -- Three-Phase Series RLC Branch37/RConn1 -- Three-Phase Series RLC Branch38/RConn1
  Bus 28/RConn2 -- Three-Phase Series RLC Branch37/RConn2 -- Three-Phase Series RLC Branch38/RConn2
  Bus 28/RConn3 -- Three-Phase Series RLC Branch38/RConn3 -- Three-Phase Series RLC Branch37/RConn3
  Three-Phase Series RLC Branch27/LConn2 -- Bus 22/LConn2
  Bus 22/LConn3 -- Three-Phase Series RLC Branch27/LConn3
  Bus 22/LConn1 -- Three-Phase Series RLC Branch27/LConn1
  Three-Phase Series RLC Branch7/LConn1 -- Bus 6/RConn1
  Three-Phase Series RLC Branch7/LConn2 -- Bus 6/RConn2
  Three-Phase Series RLC Branch7/LConn3 -- Bus 6/RConn3
  Three-Phase Series RLC Branch33/RConn1 -- Bus 27/LConn1
  Three-Phase Series RLC Branch33/RConn2 -- Bus 27/LConn2
  Three-Phase Series RLC Branch33/RConn3 -- Bus 27/LConn3
